simulink model "IEEE39_IBR_FrequencyControl_Fullversion_2023a"  (R2023a)
settings: Solver=VariableStepAuto  StartTime=0.0  StopTime=30  RelTol=1e-3
InitFcn:
  | IEEE39data_FrencyControl_full_Opensource;
undefined symbols (not defined in the file): alpha, c, eps_ps, eps_u, Fref, IBR_data, line, Sbase, t_start_disturbance, t_startcontrol, Vbase
libraries: spsThreePhaseVIMeasurementLib x61, spsThreePhasePISectionLineLib x34, spsControlledVoltageSourceLib x33, spsabctodq0Lib x33, powerlib_extras x27, spsPLL3phLib x26, spsGroundLib x22, spsThreePhaseSeriesRLCBranchLib x22, spsThreePhaseParallelRLCLoadLib x19, slpidlib x14, spsMeanLib x11, spsdq0toabcLib x11
(part 6 of 6)

== system IEEE39_IBR_FrequencyControl_Fullversion_2023a/GFM2/PV_PQ3/Freq_Droop/Subsystem1/Subsystem ==
  Dw : Inport
  w : Inport  Port=2
  Add1 : Sum
  Add2 : Sum  Inputs=+++
  Add3 : Sum  Inputs=-+
  Gain : Gain  Gain=eps_u
  Gain1 : Gain  Gain=eps_ps
  Gain2 : Gain  Gain=c(9)
  Gain3 : Gain  Gain=alpha
  Integrator : Integrator  ExternalReset=rising  ZeroCross=off
  Integrator1 : Integrator  ExternalReset=rising  ZeroCross=off
  Saturation : Saturate  UpperLimit=IBR_data(9,6)-IBR_data(9,10)  LowerLimit=IBR_data(9,6)-IBR_data(9,9)
  Step : Step  Time=3  SampleTime=0
  Step1 : Step  Time=3  SampleTime=0
  delatPset : Outport
  wires:
  w/1 -> Add2/3
  Gain2/1 -> Add2/1
  Integrator1/1 -> delatPset/1, Add3/1, Add1/1, Gain2/1
  Step/1 -> Integrator1/2
  Step1/1 -> Integrator/2
  Integrator/1 -> Gain/1
  Gain/1 -> Add2/2
  Dw/1 -> Integrator/1
  Gain1/1 -> Integrator1/1
  Add2/1 -> Gain3/1
  Gain3/1 -> Add1/2
  Add1/1 -> Saturation/1
  Saturation/1 -> Add3/2
  Add3/1 -> Gain1/1

== system IEEE39_IBR_FrequencyControl_Fullversion_2023a/GFM2/PV_PQ3/V//F/UIcontrol/wC ==
  ed : Inport
  w : Inport  Port=2
  C : Inport  Port=3
  eq : Inport  Port=4
  Product1 : Product  Inputs=3
  Product2 : Product  Inputs=3
  wC ed : Outport  VectorParamsAs1DForOutWhenUnconnected=off
  wC eq : Outport  Port=2  VectorParamsAs1DForOutWhenUnconnected=off
  wires:
  C/1 -> Product1/3, Product2/2
  Product1/1 -> wC ed/1
  w/1 -> Product1/2, Product2/1
  ed/1 -> Product1/1
  eq/1 -> Product2/3
  Product2/1 -> wC eq/1

== system IEEE39_IBR_FrequencyControl_Fullversion_2023a/GFM2/PV_PQ3/V//F/UIcontrol/wC1 ==
  id : Inport
  w : Inport  Port=2
  L : Inport  Port=3
  iq : Inport  Port=4
  Product1 : Product  Inputs=***
  Product2 : Product  Inputs=***
  wL id : Outport  VectorParamsAs1DForOutWhenUnconnected=off
  wL iq : Outport  Port=2  VectorParamsAs1DForOutWhenUnconnected=off
  wires:
  L/1 -> Product1/3, Product2/2
  Product1/1 -> wL id/1
  w/1 -> Product1/2, Product2/1
  id/1 -> Product1/1
  iq/1 -> Product2/3
  Product2/1 -> wL iq/1

== system IEEE39_IBR_FrequencyControl_Fullversion_2023a/GFM3/PV_PQ3/Freq_Droop/Subsystem1/Subsystem ==
  Dw : Inport
  w : Inport  Port=2
  Add1 : Sum
  Add2 : Sum  Inputs=+++
  Add3 : Sum  Inputs=-+
  Gain : Gain  Gain=eps_u
  Gain1 : Gain  Gain=eps_ps
  Gain2 : Gain  Gain=c(8)
  Gain3 : Gain  Gain=alpha
  Integrator : Integrator  ExternalReset=rising  ZeroCross=off
  Integrator1 : Integrator  ExternalReset=rising  ZeroCross=off
  Saturation : Saturate  UpperLimit=IBR_data(8,6)-IBR_data(8,10)  LowerLimit=IBR_data(8,6)-IBR_data(8,9)
  Step : Step  Time=3  SampleTime=0
  Step1 : Step  Time=3  SampleTime=0
  delatPset : Outport
  wires:
  w/1 -> Add2/3
  Gain2/1 -> Add2/1
  Integrator1/1 -> delatPset/1, Add3/1, Add1/1, Gain2/1
  Step/1 -> Integrator1/2
  Step1/1 -> Integrator/2
  Integrator/1 -> Gain/1
  Gain/1 -> Add2/2
  Dw/1 -> Integrator/1
  Gain1/1 -> Integrator1/1
  Add2/1 -> Gain3/1
  Gain3/1 -> Add1/2
  Add1/1 -> Saturation/1
  Saturation/1 -> Add3/2
  Add3/1 -> Gain1/1

== system IEEE39_IBR_FrequencyControl_Fullversion_2023a/GFM3/PV_PQ3/V//F/UIcontrol/wC ==
  ed : Inport
  w : Inport  Port=2
  C : Inport  Port=3
  eq : Inport  Port=4
  Product1 : Product  Inputs=3
  Product2 : Product  Inputs=3
  wC ed : Outport  VectorParamsAs1DForOutWhenUnconnected=off
  wC eq : Outport  Port=2  VectorParamsAs1DForOutWhenUnconnected=off
  wires:
  C/1 -> Product1/3, Product2/2
  Product1/1 -> wC ed/1
  w/1 -> Product1/2, Product2/1
  ed/1 -> Product1/1
  eq/1 -> Product2/3
  Product2/1 -> wC eq/1

== system IEEE39_IBR_FrequencyControl_Fullversion_2023a/GFM3/PV_PQ3/V//F/UIcontrol/wC1 ==
  id : Inport
  w : Inport  Port=2
  L : Inport  Port=3
  iq : Inport  Port=4
  Product1 : Product  Inputs=***
  Product2 : Product  Inputs=***
  wL id : Outport  VectorParamsAs1DForOutWhenUnconnected=off
  wL iq : Outport  Port=2  VectorParamsAs1DForOutWhenUnconnected=off
  wires:
  L/1 -> Product1/3, Product2/2
  Product1/1 -> wL id/1
  w/1 -> Product1/2, Product2/1
  id/1 -> Product1/1
  iq/1 -> Product2/3
  Product2/1 -> wL iq/1

== system IEEE39_IBR_FrequencyControl_Fullversion_2023a/GFM4/PV_PQ3/Freq_Droop/Subsystem1/Subsystem ==
  Dw : Inport
  w : Inport  Port=2
  Add1 : Sum
  Add2 : Sum  Inputs=+++
  Add3 : Sum  Inputs=-+
  Gain : Gain  Gain=eps_u
  Gain1 : Gain  Gain=eps_ps
  Gain2 : Gain  Gain=c(7)
  Gain3 : Gain  Gain=alpha
  Integrator : Integrator  ExternalReset=rising  ZeroCross=off
  Integrator1 : Integrator  ExternalReset=rising  ZeroCross=off
  Saturation : Saturate  UpperLimit=IBR_data(7,6)-IBR_data(7,10)  LowerLimit=IBR_data(7,6)-IBR_data(7,9)
  Step : Step  Time=3  SampleTime=0
  Step1 : Step  Time=3  SampleTime=0
  delatPset : Outport
  wires:
  w/1 -> Add2/3
  Gain2/1 -> Add2/1
  Integrator1/1 -> delatPset/1, Add3/1, Add1/1, Gain2/1
  Step/1 -> Integrator1/2
  Step1/1 -> Integrator/2
  Integrator/1 -> Gain/1
  Gain/1 -> Add2/2
  Dw/1 -> Integrator/1
  Gain1/1 -> Integrator1/1
  Add2/1 -> Gain3/1
  Gain3/1 -> Add1/2
  Add1/1 -> Saturation/1
  Saturation/1 -> Add3/2
  Add3/1 -> Gain1/1

== system IEEE39_IBR_FrequencyControl_Fullversion_2023a/GFM4/PV_PQ3/V//F/UIcontrol/wC ==
  ed : Inport
  w : Inport  Port=2
  C : Inport  Port=3
  eq : Inport  Port=4
  Product1 : Product  Inputs=3
  Product2 : Product  Inputs=3
  wC ed : Outport  VectorParamsAs1DForOutWhenUnconnected=off
  wC eq : Outport  Port=2  VectorParamsAs1DForOutWhenUnconnected=off
  wires:
  C/1 -> Product1/3, Product2/2
  Product1/1 -> wC ed/1
  w/1 -> Product1/2, Product2/1
  ed/1 -> Product1/1
  eq/1 -> Product2/3
  Product2/1 -> wC eq/1

== system IEEE39_IBR_FrequencyControl_Fullversion_2023a/GFM4/PV_PQ3/V//F/UIcontrol/wC1 ==
  id : Inport
  w : Inport  Port=2
  L : Inport  Port=3
  iq : Inport  Port=4
  Product1 : Product  Inputs=***
  Product2 : Product  Inputs=***
  wL id : Outport  VectorParamsAs1DForOutWhenUnconnected=off
  wL iq : Outport  Port=2  VectorParamsAs1DForOutWhenUnconnected=off
  wires:
  L/1 -> Product1/3, Product2/2
  Product1/1 -> wL id/1
  w/1 -> Product1/2, Product2/1
  id/1 -> Product1/1
  iq/1 -> Product2/3
  Product2/1 -> wL iq/1
